simulink model "35 Bus Network Electricity Transmission Model"  (R2023b)
settings: Solver=VariableStepAuto  StartTime=0.0  StopTime=1  RelTol=1e-3
model workspace (MAT data in the model file):
  T_set = 0.0001
  Tp = 5e-05
undefined symbols (not defined in the file): D1, D11, Delta, DiscIntNeverNeededParam
libraries: spsSeriesRLCBranchLib x57, spsLoadFlowBusLib x35, spsThreePhaseSeriesRLCLoadLib x28, spsThreePhaseTransformerTwoWindingsLib x22, spsDistributedParametersLineLib x22, spsGenericPowerSystemStabilizerLib x20, spsThreePhaseVIMeasurementLib x14, spsSynchronousMachinepuStandardLib x10, spsExcitationSystemLib x10, spsHydraulicTurbineandGovernorLib x10, spsFourierLib x8, spsMeanLib x8
(part 7 of 8)

== system 35 Bus Network Electricity Transmission Model/400 kV Solar Farm/VSC Control/Current Regulator ==
  note: harmonic filter neglected
  note: Vd_mes + Id*R - Iq*L + deriv(Id)*L= Vd_conv
  note: Vq_mes + Id*L + Iq*R + deriv(Iq)*L= Vq_conv
  note: Current Regulator
      | (with feedforward)
  note: Sign Convention: Current going out of the converter = positive current
  note: Iq positive --> The converter absorbs reactive power ("Inductive mode") = Reactive Power Q negative
  note: Id positive --> The converter generates active power ("Inverter mode") = Active Power P positive
  note: Ltot = Lxfo + Lchoke
      | Rtot = Rxfo + Rchoke
  note: (Vd_prim - Vd_conv) ~= + Iq * Ltot
  note: (Vq_prim - Vq_conv) ~ = - Id * Ltot
  note: For Ltot >> Rtot :
  VdVq_mes : Inport  PortDimensions=2
  IdIq_mes : Inport  Port=2  PortDimensions=2
  IdIq_ref : Inport  Port=3  PortDimensions=2
  Add1 : Sum  Inputs=++-
  Add2 : Sum
  Add3 : Sum  Inputs=+++
  Demux : Demux  Outputs=2
  Demux1 : Demux  Outputs=2
  Ltot_pu1 : Gain  Gain=Ltot_pu  SaturateOnIntegerOverflow=on  OutDataTypeStr=Inherit: Same as input  ParamDataTypeStr=Inherit: Same as input
  Ltot_pu2 : Gain  Gain=Ltot_pu  SaturateOnIntegerOverflow=on  OutDataTypeStr=Inherit: Same as input  ParamDataTypeStr=Inherit: Same as input
  Mux : Mux  Inputs=2
  PI : slpidlib/PID Controller  Controller=PI  Form=Parallel  TimeDomain=Discrete-time  UseExternalTs=off  SampleTime=Ts  IntegratorMethod=Forward Euler  FilterMethod=Forward Euler  ControllerParametersSource=internal  P=Kp_Ireg  I=Ki_Ireg  UseKiTs=off  D=0  N=100  UseFilter=on  TunerSelectOption=Transfer Function Based (PID Tuner App)  InitialConditionSource=internal  InitialConditionForIntegrator=0  InitialConditionForFilter=0  DifferentiatorICPrevScaledInput=0  ExternalReset=none  TrackingMode=off  Kt=1  LimitOutput=on  SatLimitsSource=internal  UpperSaturationLimit=2  LowerSaturationLimit=-2  LinearizeAsGain=off  AntiWindupMode=none  Kb=1  LimitIntegrator=off  UpperIntegratorSaturationLimit=inf  LowerIntegratorSaturationLimit=-inf  POutMin=[]  POutMax=[]  IOutMin=[]  IOutMax=[]  DOutMin=[]  DOutMax=[]  NOutMin=[]  NOutMax=[]  SumOutMin=[]  SumOutMax=[]  SaturationOutMin=[]  SaturationOutMax=[]  PParamMin=[]  PParamMax=[]  IParamMin=[]  IParamMax=[]  DParamMin=[]  DParamMax=[]  NParamMin=[]  NParamMax=[]  KbParamMin=[]  KbParamMax=[]  KtParamMin=[]  KtParamMax=[]  KbOutMin=[]  KbOutMax=[]  KtOutMin=[]  KtOutMax=[]  IntegratorOutMin=[]  IntegratorOutMax=[]  FilterOutMin=[]  FilterOutMax=[]  SumI1OutMin=[]  SumI1OutMax=[]  SumI2OutMin=[]  SumI2OutMax=[]  SumI3OutMin=[]  SumI3OutMax=[]  SumI4OutMin=[]  SumI4OutMax=[]  SumDOutMin=[]  SumDOutMax=[]  DifferentiatorOutMin=[]  DifferentiatorOutMax=[]  FilterDiffOutCoefMin=[]  FilterDiffOutCoefMax=[]  ReciprocalOutMin=[]  ReciprocalOutMax=[]  SumDenOutMin=[]  SumDenOutMax=[]  SumNumOutMin=[]  SumNumOutMax=[]  DivideOutMin=[]  DivideOutMax=[]  UdiffTsProdOutMin=[]  UdiffTsProdOutMax=[]  NTsProdOutMin=[]  NTsProdOutMax=[]  UintegralTsProdOutMin=[]  UintegralTsProdOutMax=[]  UngainTsProdOutMin=[]  UngainTsProdOutMax=[]  ClampingZeroOutDataTypeStr=Inherit: Inherit via back propagation  ClampingZeroOutMin=[]  ClampingZeroOutMax=[]  FilterDenConstantOutDataTypeStr=Inherit: Inherit via back propagation  FilterDenConstantOutMin=[]  FilterDenConstantOutMax=[]  PCopyOutDataTypeStr=Inherit: Inherit via back propagation  PCopyOutMin=[]  PCopyOutMax=[]  NCopyOutDataTypeStr=Inherit: Inherit via back propagation  NCopyOutMin=[]  NCopyOutMax=[]  IntegratorContinuousStateAttributes=''  IntegratorStateMustResolveToSignalObject=off  IntegratorRTWStateStorageClass=Auto  FilterContinuousStateAttributes=''  FilterStateMustResolveToSignalObject=off  FilterRTWStateStorageClass=Auto  ParallelPVariant=InternalParameters  IdealPVariant=Disabled  IVariant=InternalParameters  DVariant=Disabled  IntegratorVariant=Discrete  SatVariant=Enabled  AWVariant=Passthrough  PCopyVariant=Disabled  TRVariant=Disabled  FdbkBlocksVariant=Forward  IdealPFdbkVariant=Disabled  SatFdbkVariant=Disabled  DerivativeFilterVariant=Disabled  NVariant=Disabled  NCopyVariant=Disabled_SignalSpec  FilterICVariant=Disabled  IntegratorICVariant=InternalICs  ExternalResetVariant=Disabled  TRSumVariant=Passthrough  SumFdbkVariant=Disabled  SumVariant=Sum_PI  TsampFilterVariant=InternalTs  TsampNgainVariant=Passthrough  TsampIntegralVariant=Disabled_SignalSpec  ExternalSaturationOutDataTypeStr=Inherit: Same as second input
  PI_Ireg1 : Scope
  Rtot_pu1 : Gain  Gain=Rtot_pu  SaturateOnIntegerOverflow=on  OutDataTypeStr=Inherit: Same as input  ParamDataTypeStr=Inherit: Same as input
  Rtot_pu5 : Gain  Gain=Rtot_pu  SaturateOnIntegerOverflow=on  OutDataTypeStr=Inherit: Same as input  ParamDataTypeStr=Inherit: Same as input
  Saturation : Saturate  UpperLimit=2  LowerLimit=-2
  Sum : Sum  Inputs=|-+
  VdVq_conv : Outport  VectorParamsAs1DForOutWhenUnconnected=off
  wires:
  Mux/1 -> PI_Ireg1/1, Add2/2
  PI/1 -> Add2/1  "PI"
  Sum/1 -> PI/1
  IdIq_ref/1 -> Sum/2, Demux1/1
  IdIq_mes/1 -> Sum/1
  Add2/1 -> Saturation/1
  Saturation/1 -> VdVq_conv/1
  VdVq_mes/1 -> Demux/1
  Demux/1 -> Add1/1
  Rtot_pu1/1 -> Add1/2
  Demux1/1 -> Rtot_pu1/1, Ltot_pu2/1
  Ltot_pu1/1 -> Add1/3
  Demux1/2 -> Ltot_pu1/1, Rtot_pu5/1
  Rtot_pu5/1 -> Add3/2
  Ltot_pu2/1 -> Add3/3
  Add1/1 -> Mux/1  "Feedforward"
  Demux/2 -> Add3/1
  Add3/1 -> Mux/2

== system 35 Bus Network Electricity Transmission Model/400 kV Solar Farm/VSC Control/PLL & Measurements ==
  Vabc_prim : Inport
  Iabc_prim : Inport  Port=2
  PLL (3ph) : spsPLL3phLib/PLL (3ph)  Fmin=45  Par_Init="[-0.57  Fnom]"  ParK=[180, 3200, 1]  TcD=Ts  MaxRateChangeFreq=12  FilterCutOffFreq=25  Ts=Ts  AGC=on
  Selector1 : Selector  InputPortWidth=3  IndexOptions=Index vector (dialog)  Indices=[1 2]  OutputSizes=1
  Selector2 : Selector  InputPortWidth=3  IndexOptions=Index vector (dialog)  Indices=[1 2]  OutputSizes=1
  Terminator : Terminator
  V->pu : Gain  Gain=1/(Vnom_prim*sqrt(2)/sqrt(3))  SaturateOnIntegerOverflow=on  OutDataTypeStr=Inherit: Same as input  ParamDataTypeStr=Inherit: Same as input
  V->pu1 : Gain  Gain=Vnom_prim*sqrt(3)/Pnom/sqrt(2)  SaturateOnIntegerOverflow=on  OutDataTypeStr=Inherit: Same as input  ParamDataTypeStr=Inherit: Same as input
  abc to dq0 : spsabctodq0Lib/abc to dq0  Alignment=90 degrees behind phase A axis
  abc to dq1 : spsabctodq0Lib/abc to dq0  Alignment=90 degrees behind phase A axis
  wt : Outport  VectorParamsAs1DForOutWhenUnconnected=off
  VdVq_prim : Outport  Port=2  VectorParamsAs1DForOutWhenUnconnected=off
  IdIq_prim : Outport  Port=3  VectorParamsAs1DForOutWhenUnconnected=off
  wires:
  V->pu1/1 -> abc to dq1/1
  V->pu/1 -> PLL (3ph)/1, abc to dq0/1
  abc to dq1/1 -> Selector1/1
  Vabc_prim/1 -> V->pu/1
  Iabc_prim/1 -> V->pu1/1
  abc to dq0/1 -> Selector2/1
  Selector2/1 -> VdVq_prim/1
  Selector1/1 -> IdIq_prim/1
  PLL (3ph)/2 -> wt/1, abc to dq1/2, abc to dq0/2
  PLL (3ph)/1 -> Terminator/1

== system 35 Bus Network Electricity Transmission Model/400 kV Solar Farm/VSC Control/Uabc_ref Generation max (m) = 1 ==
  note: (Correction for transformer
      |  D1 connection)
  note: (Correction for delai of Ts_Control)
  wt : Inport
  VdVq_conv : Inport  Port=2
  Add1 : Sum  Inputs=++++
  Add2 : Sum
  Complex to Magnitude-Angle : ComplexToMagnitudeAngle
  Constant : Constant  Value=-pi/6
  Constant1 : Constant  Value=Vnom_dc
  Constant2 : Constant  Value="[ 0  -2*pi/3  2*pi/3  ]"
  Constant3 : Constant  Value=Vnom_sec*sqrt(2)/sqrt(3)
  Constant4 : Constant  Value=Ts*Fnom*(2*pi)
  Demux1 : Demux  Outputs=2
  Gain1 : Gain  Gain=1/2
  Product : Product  Inputs=*/  RndMeth=Zero
  Product1 : Product  Inputs=*/  RndMeth=Zero
  Product2 : Product  Inputs=**  RndMeth=Zero
  Real-Imag to Complex : RealImagToComplex
  Saturation : Saturate  UpperLimit=1  LowerLimit=0
  Trigonometric Function : Trigonometry
  Uabc_ref : Outport  VectorParamsAs1DForOutWhenUnconnected=off
  wires:
  Complex to Magnitude-Angle/1 -> Saturation/1
  Constant1/1 -> Gain1/1
  VdVq_conv/1 -> Product1/1
  Product1/1 -> Demux1/1
  Gain1/1 -> Product/1
  Real-Imag to Complex/1 -> Complex to Magnitude-Angle/1
  Demux1/1 -> Real-Imag to Complex/1
  Demux1/2 -> Real-Imag to Complex/2
  Constant2/1 -> Add1/2
  Constant/1 -> Add1/3
  Constant3/1 -> Product/2
  Product/1 -> Product1/2
  Complex to Magnitude-Angle/2 -> Add2/1
  Add1/1 -> Add2/2
  Add2/1 -> Trigonometric Function/1
  Saturation/1 -> Product2/1
  Trigonometric Function/1 -> Product2/2
  Product2/1 -> Uabc_ref/1
  wt/1 -> Add1/1
  Constant4/1 -> Add1/4

== system 35 Bus Network Electricity Transmission Model/400 kV Solar Farm/VSC Control/VDC Regulator ==
  Vdc_mes : Inport  PortDimensions=1
  Vdc_ref : Inport  Port=2  PortDimensions=1
  PI : slpidlib/PID Controller  Controller=PI  Form=Parallel  TimeDomain=Discrete-time  UseExternalTs=off  SampleTime=Ts  IntegratorMethod=Trapezoidal  FilterMethod=Forward Euler  ControllerParametersSource=internal  P=Kp_VDCreg  I=Ki_VDCreg  UseKiTs=off  D=0  N=100  UseFilter=on  TunerSelectOption=Transfer Function Based (PID Tuner App)  InitialConditionSource=internal  InitialConditionForIntegrator=0  InitialConditionForFilter=0  DifferentiatorICPrevScaledInput=0  ExternalReset=none  TrackingMode=off  Kt=1  LimitOutput=on  SatLimitsSource=internal  UpperSaturationLimit=1.5  LowerSaturationLimit=-1.5  LinearizeAsGain=off  AntiWindupMode=none  Kb=1  LimitIntegrator=off  UpperIntegratorSaturationLimit=inf  LowerIntegratorSaturationLimit=-inf  POutMin=[]  POutMax=[]  IOutMin=[]  IOutMax=[]  DOutMin=[]  DOutMax=[]  NOutMin=[]  NOutMax=[]  SumOutMin=[]  SumOutMax=[]  SaturationOutMin=[]  SaturationOutMax=[]  PParamMin=[]  PParamMax=[]  IParamMin=[]  IParamMax=[]  DParamMin=[]  DParamMax=[]  NParamMin=[]  NParamMax=[]  KbParamMin=[]  KbParamMax=[]  KtParamMin=[]  KtParamMax=[]  KbOutMin=[]  KbOutMax=[]  KtOutMin=[]  KtOutMax=[]  IntegratorOutMin=[]  IntegratorOutMax=[]  FilterOutMin=[]  FilterOutMax=[]  SumI1OutMin=[]  SumI1OutMax=[]  SumI2OutMin=[]  SumI2OutMax=[]  SumI3OutMin=[]  SumI3OutMax=[]  SumI4OutMin=[]  SumI4OutMax=[]  SumDOutMin=[]  SumDOutMax=[]  DifferentiatorOutMin=[]  DifferentiatorOutMax=[]  FilterDiffOutCoefMin=[]  FilterDiffOutCoefMax=[]  ReciprocalOutMin=[]  ReciprocalOutMax=[]  SumDenOutMin=[]  SumDenOutMax=[]  SumNumOutMin=[]  SumNumOutMax=[]  DivideOutMin=[]  DivideOutMax=[]  UdiffTsProdOutMin=[]  UdiffTsProdOutMax=[]  NTsProdOutMin=[]  NTsProdOutMax=[]  UintegralTsProdOutMin=[]  UintegralTsProdOutMax=[]  UngainTsProdOutMin=[]  UngainTsProdOutMax=[]  ClampingZeroOutDataTypeStr=Inherit: Inherit via back propagation  ClampingZeroOutMin=[]  ClampingZeroOutMax=[]  FilterDenConstantOutDataTypeStr=Inherit: Inherit via back propagation  FilterDenConstantOutMin=[]  FilterDenConstantOutMax=[]  PCopyOutDataTypeStr=Inherit: Inherit via back propagation  PCopyOutMin=[]  PCopyOutMax=[]  NCopyOutDataTypeStr=Inherit: Inherit via back propagation  NCopyOutMin=[]  NCopyOutMax=[]  IntegratorContinuousStateAttributes=''  IntegratorStateMustResolveToSignalObject=off  IntegratorRTWStateStorageClass=Auto  FilterContinuousStateAttributes=''  FilterStateMustResolveToSignalObject=off  FilterRTWStateStorageClass=Auto  ParallelPVariant=InternalParameters  IdealPVariant=Disabled  IVariant=InternalParameters  DVariant=Disabled  IntegratorVariant=Discrete  SatVariant=Enabled  AWVariant=Passthrough  PCopyVariant=Disabled  TRVariant=Disabled  FdbkBlocksVariant=Forward  IdealPFdbkVariant=Disabled  SatFdbkVariant=Disabled  DerivativeFilterVariant=Disabled  NVariant=Disabled  NCopyVariant=Disabled_SignalSpec  FilterICVariant=Disabled  IntegratorICVariant=InternalICs  ExternalResetVariant=Disabled  TRSumVariant=Passthrough  SumFdbkVariant=Disabled  SumVariant=Sum_PI  TsampFilterVariant=InternalTs  TsampNgainVariant=Passthrough  TsampIntegralVariant=Disabled_SignalSpec  ExternalSaturationOutDataTypeStr=Inherit: Same as second input
  Rtot_pu3 : Gain  Gain=1/Vnom_dc  SaturateOnIntegerOverflow=on  OutDataTypeStr=Inherit: Same as input  ParamDataTypeStr=Inherit: Same as input
  Sum : Sum  Inputs=|+-
  Id_ref : Outport  SampleTime=Ts  InitialOutput=0  VectorParamsAs1DForOutWhenUnconnected=off
  wires:
  Sum/1 -> Rtot_pu3/1
  Vdc_mes/1 -> Sum/1
  Vdc_ref/1 -> Sum/2
  Rtot_pu3/1 -> PI/1
  PI/1 -> Id_ref/1

== system 35 Bus Network Electricity Transmission Model/North Network/Regulators 7/Turbine and Excitation Regulators ==
  pref : Inport
  w : Inport  Port=2
  Pe 0 : Inport  Port=3
  Vref : Inport  Port=4
  Vm : Inport  Port=5
  Add : Sum  Inputs=+-
  Complex to Real-Imag : ComplexToRealImag
  Excitation System : spsExcitationSystemLib/Excitation System  tr=20e-3  reg=[ 300, 0.001 ]  exc=[ 1, 0 ]  tgr=[ 0, 0 ]  damp=[ 0.001, 0.1 ]  sat=[ 0, 0 ]  lim=[ -11.5, 11.5, 0 ]  v0="[1.0  1.28]"
      settings: LibrarySourceBlock=sps_lib/Electrical Machines/Synchronous Machine Control/Excitation System
  Hydraulic Turbine and Governor : spsHydraulicTurbineandGovernorLib/Hydraulic Turbine and Governor  sm="[ 10/3  0.07 ]"  gate="[  0.01  0.97518  -0.1  0.1 ]"  reg="[  0.05  1.163  0.105  0  0.01  ]"  hyd="[  0  2.67  ]"  dref=0  po=0.7516
      settings: LibrarySourceBlock=|
      | sps_lib/Electrical Machines/Synchronous Machine Control/Hydraulic Turbine
      | and Governor
  Stabilitator : Subsystem
  Terminator : Terminator
  wref : Constant
  wref1 : Constant
  Pm : Outport
  Vf : Outport  Port=2
  wires:
  pref/1 -> Hydraulic Turbine and Governor/2
  Complex to Real-Imag/2 -> Excitation System/3
  wref/1 -> Hydraulic Turbine and Governor/1
  Add/1 -> Stabilitator/3(dw), Hydraulic Turbine and Governor/5
  Vm/1 -> Complex to Real-Imag/1
  Pe 0/1 -> Stabilitator/2(Pe), Hydraulic Turbine and Governor/4
  Hydraulic Turbine and Governor/2 -> Terminator/1
  Stabilitator/1(Out1) -> Excitation System/4
  w/1 -> Add/1, Hydraulic Turbine and Governor/3
  Excitation System/1 -> Vf/1
  Hydraulic Turbine and Governor/1 -> Pm/1, Stabilitator/1(Pm)
  Vref/1 -> Excitation System/1
  wref1/1 -> Add/2
  Complex to Real-Imag/1 -> Excitation System/2

== system 35 Bus Network Electricity Transmission Model/North Network/Regulators 8/Turbine and Excitation Regulators ==
  pref : Inport
  w : Inport  Port=2
  Pe 0 : Inport  Port=3
  Vref : Inport  Port=4
  Vm : Inport  Port=5
  Add : Sum  Inputs=+-
  Complex to Real-Imag : ComplexToRealImag
  Excitation System : spsExcitationSystemLib/Excitation System  tr=20e-3  reg=[ 300, 0.001 ]  exc=[ 1, 0 ]  tgr=[ 0, 0 ]  damp=[ 0.001, 0.1 ]  sat=[ 0, 0 ]  lim=[ -11.5, 11.5, 0 ]  v0="[1.0  1.28]"
      settings: LibrarySourceBlock=sps_lib/Electrical Machines/Synchronous Machine Control/Excitation System
  Hydraulic Turbine and Governor : spsHydraulicTurbineandGovernorLib/Hydraulic Turbine and Governor  sm="[ 10/3  0.07 ]"  gate="[  0.01  0.97518  -0.1  0.1 ]"  reg="[  0.05  1.163  0.105  0  0.01  ]"  hyd="[  0  2.67  ]"  dref=0  po=0.7516
      settings: LibrarySourceBlock=|
      | sps_lib/Electrical Machines/Synchronous Machine Control/Hydraulic Turbine
      | and Governor
  Stabilitator : Subsystem
  Terminator : Terminator
  wref : Constant
  wref1 : Constant
  Pm : Outport
  Vf : Outport  Port=2
  wires:
  pref/1 -> Hydraulic Turbine and Governor/2
  Complex to Real-Imag/2 -> Excitation System/3
  wref/1 -> Hydraulic Turbine and Governor/1
  Add/1 -> Stabilitator/3(dw), Hydraulic Turbine and Governor/5
  Vm/1 -> Complex to Real-Imag/1
  Pe 0/1 -> Stabilitator/2(Pe), Hydraulic Turbine and Governor/4
  Hydraulic Turbine and Governor/2 -> Terminator/1
  Stabilitator/1(Out1) -> Excitation System/4
  w/1 -> Add/1, Hydraulic Turbine and Governor/3
  Excitation System/1 -> Vf/1
  Hydraulic Turbine and Governor/1 -> Pm/1, Stabilitator/1(Pm)
  Vref/1 -> Excitation System/1
  wref1/1 -> Add/2
  Complex to Real-Imag/1 -> Excitation System/2

== system 35 Bus Network Electricity Transmission Model/North Network/Regulators 9/Turbine and Excitation Regulators ==
  pref : Inport
  w : Inport  Port=2
  Pe 0 : Inport  Port=3
  Vref : Inport  Port=4
  Vm : Inport  Port=5
  Add : Sum  Inputs=+-
  Complex to Real-Imag : ComplexToRealImag
  Excitation System : spsExcitationSystemLib/Excitation System  tr=20e-3  reg=[ 300, 0.001 ]  exc=[ 1, 0 ]  tgr=[ 0, 0 ]  damp=[ 0.001, 0.1 ]  sat=[ 0, 0 ]  lim=[ -11.5, 11.5, 0 ]  v0="[1.0  1.28]"
      settings: LibrarySourceBlock=sps_lib/Electrical Machines/Synchronous Machine Control/Excitation System
  Hydraulic Turbine and Governor : spsHydraulicTurbineandGovernorLib/Hydraulic Turbine and Governor  sm="[ 10/3  0.07 ]"  gate="[  0.01  0.97518  -0.1  0.1 ]"  reg="[  0.05  1.163  0.105  0  0.01  ]"  hyd="[  0  2.67  ]"  dref=0  po=0.7516
      settings: LibrarySourceBlock=|
      | sps_lib/Electrical Machines/Synchronous Machine Control/Hydraulic Turbine
      | and Governor
  Stabilitator : Subsystem
  Terminator : Terminator
  wref : Constant
  wref1 : Constant
  Pm : Outport
  Vf : Outport  Port=2
  wires:
  pref/1 -> Hydraulic Turbine and Governor/2
  Complex to Real-Imag/2 -> Excitation System/3
  wref/1 -> Hydraulic Turbine and Governor/1
  Add/1 -> Stabilitator/3(dw), Hydraulic Turbine and Governor/5
  Vm/1 -> Complex to Real-Imag/1
  Pe 0/1 -> Stabilitator/2(Pe), Hydraulic Turbine and Governor/4
  Hydraulic Turbine and Governor/2 -> Terminator/1
  Stabilitator/1(Stab) -> Excitation System/4
  w/1 -> Add/1, Hydraulic Turbine and Governor/3
  Excitation System/1 -> Vf/1
  Hydraulic Turbine and Governor/1 -> Pm/1, Stabilitator/1(Pm)
  Vref/1 -> Excitation System/1
  wref1/1 -> Add/2
  Complex to Real-Imag/1 -> Excitation System/2

== system 35 Bus Network Electricity Transmission Model/Regulators 10/Turbine and Excitation Regulators/Stabilitator ==
  Pm : Inport
  Pe : Inport  Port=2
  dw : Inport  Port=3
  Add1 : Sum  Inputs=+-
  Generic Power System Stabilizer : spsGenericPowerSystemStabilizerLib/Generic Power System Stabilizer  Tsensor=30e-3  K=20  Twashout=2  Tleadlag1=[50e-3 20e-3]  Tleadlag2=[3 5.4]  VSlimits=[-0.15 0.15]  Vinit=0  Plot_On=off  MagdB_On=on  FreqRange=logspace(-2,2,500)
      settings: LibrarySourceBlock=|
      | sps_lib/Electrical Machines/Synchronous Machine Control/Generic
      | Power System Stabilizer
  Generic Power System Stabilizer1 : spsGenericPowerSystemStabilizerLib/Generic Power System Stabilizer  Tsensor=30e-3  K=20  Twashout=2  Tleadlag1=[50e-3 20e-3]  Tleadlag2=[3 5.4]  VSlimits=[-0.15 0.15]  Vinit=0  Plot_On=off  MagdB_On=on  FreqRange=logspace(-2,2,500)
      settings: LibrarySourceBlock=|
      | sps_lib/Electrical Machines/Synchronous Machine Control/Generic
      | Power System Stabilizer
  Ground : Ground
  Multiport Switch : MultiPortSwitch  DiagnosticForDefault=None  SaturateOnIntegerOverflow=off  InputSameDT=off
  Out1 : Outport
  wires:
  Pm/1 -> Add1/1
  Generic Power System Stabilizer1/1 -> Multiport Switch/4
  Pe/1 -> Add1/2
  Add1/1 -> Generic Power System Stabilizer/1
  Generic Power System Stabilizer/1 -> Multiport Switch/3
  dw/1 -> Generic Power System Stabilizer1/1
  Ground/1 -> Multiport Switch/2
  [PSS_modes] -> Multiport Switch/1
  Multiport Switch/1 -> Out1/1

== system 35 Bus Network Electricity Transmission Model/South Network/Regulators 1/Turbine and Excitation Regulators ==
  pref : Inport
  w : Inport  Port=2
  Pe 0 : Inport  Port=3
  Vref : Inport  Port=4
  Vm : Inport  Port=5
  Add : Sum  Inputs=+-
  Complex to Real-Imag : ComplexToRealImag
  Excitation System : spsExcitationSystemLib/Excitation System  tr=20e-3  reg=[ 300, 0.001 ]  exc=[ 1, 0 ]  tgr=[ 0, 0 ]  damp=[ 0.001, 0.1 ]  sat=[ 0, 0 ]  lim=[ -11.5, 11.5, 0 ]  v0="[1.0  1.28]"
      settings: LibrarySourceBlock=sps_lib/Electrical Machines/Synchronous Machine Control/Excitation System
  Hydraulic Turbine and Governor : spsHydraulicTurbineandGovernorLib/Hydraulic Turbine and Governor  sm="[ 10/3  0.07 ]"  gate="[  0.01  0.97518  -0.1  0.1 ]"  reg="[  0.05  1.163  0.105  0  0.01  ]"  hyd="[  0  2.67  ]"  dref=0  po=0.7516
      settings: LibrarySourceBlock=|
      | sps_lib/Electrical Machines/Synchronous Machine Control/Hydraulic Turbine
      | and Governor
  Stabilitator : Subsystem
  Terminator : Terminator
  wref : Constant
  wref1 : Constant
  Pm : Outport
  Vf : Outport  Port=2
  wires:
  pref/1 -> Hydraulic Turbine and Governor/2
  Complex to Real-Imag/2 -> Excitation System/3
  wref/1 -> Hydraulic Turbine and Governor/1
  Add/1 -> Stabilitator/3(dw), Hydraulic Turbine and Governor/5
  Vm/1 -> Complex to Real-Imag/1
  Pe 0/1 -> Stabilitator/2(Pe), Hydraulic Turbine and Governor/4
  Hydraulic Turbine and Governor/2 -> Terminator/1
  Stabilitator/1(Out1) -> Excitation System/4
  w/1 -> Add/1, Hydraulic Turbine and Governor/3
  Excitation System/1 -> Vf/1
  Hydraulic Turbine and Governor/1 -> Pm/1, Stabilitator/1(Pm)
  Vref/1 -> Excitation System/1
  wref1/1 -> Add/2
  Complex to Real-Imag/1 -> Excitation System/2

== system 35 Bus Network Electricity Transmission Model/South Network/Regulators 2/Turbine and Excitation Regulators ==
  pref : Inport
  w : Inport  Port=2
  Pe 0 : Inport  Port=3
  Vref : Inport  Port=4
  Vm : Inport  Port=5
  Add : Sum  Inputs=+-
  Complex to Real-Imag : ComplexToRealImag
  Excitation System : spsExcitationSystemLib/Excitation System  tr=20e-3  reg=[ 300, 0.001 ]  exc=[ 1, 0 ]  tgr=[ 0, 0 ]  damp=[ 0.001, 0.1 ]  sat=[ 0, 0 ]  lim=[ -11.5, 11.5, 0 ]  v0="[1.0  1.28]"
      settings: LibrarySourceBlock=sps_lib/Electrical Machines/Synchronous Machine Control/Excitation System
  Hydraulic Turbine and Governor : spsHydraulicTurbineandGovernorLib/Hydraulic Turbine and Governor  sm="[ 10/3  0.07 ]"  gate="[  0.01  0.97518  -0.1  0.1 ]"  reg="[  0.05  1.163  0.105  0  0.01  ]"  hyd="[  0  2.67  ]"  dref=0  po=0.7516
      settings: LibrarySourceBlock=|
      | sps_lib/Electrical Machines/Synchronous Machine Control/Hydraulic Turbine
      | and Governor
  Stabilitator : Subsystem
  Terminator : Terminator
  wref : Constant
  wref1 : Constant
  Pm : Outport
  Vf : Outport  Port=2
  wires:
  pref/1 -> Hydraulic Turbine and Governor/2
  Complex to Real-Imag/2 -> Excitation System/3
  wref/1 -> Hydraulic Turbine and Governor/1
  Add/1 -> Stabilitator/3(dw), Hydraulic Turbine and Governor/5
  Vm/1 -> Complex to Real-Imag/1
  Pe 0/1 -> Stabilitator/2(Pe), Hydraulic Turbine and Governor/4
  Hydraulic Turbine and Governor/2 -> Terminator/1
  Stabilitator/1(Out1) -> Excitation System/4
  w/1 -> Add/1, Hydraulic Turbine and Governor/3
  Excitation System/1 -> Vf/1
  Hydraulic Turbine and Governor/1 -> Pm/1, Stabilitator/1(Pm)
  Vref/1 -> Excitation System/1
  wref1/1 -> Add/2
  Complex to Real-Imag/1 -> Excitation System/2

== system 35 Bus Network Electricity Transmission Model/South Network/Regulators 3/Turbine and Excitation Regulators ==
  pref : Inport
  w : Inport  Port=2
  Pe 0 : Inport  Port=3
  Vref : Inport  Port=4
  Vm : Inport  Port=5
  Add : Sum  Inputs=+-
  Complex to Real-Imag : ComplexToRealImag
  Excitation System : spsExcitationSystemLib/Excitation System  tr=20e-3  reg=[ 300, 0.001 ]  exc=[ 1, 0 ]  tgr=[ 0, 0 ]  damp=[ 0.001, 0.1 ]  sat=[ 0, 0 ]  lim=[ -11.5, 11.5, 0 ]  v0="[1.0  1.28]"
      settings: LibrarySourceBlock=sps_lib/Electrical Machines/Synchronous Machine Control/Excitation System
  Hydraulic Turbine and Governor : spsHydraulicTurbineandGovernorLib/Hydraulic Turbine and Governor  sm="[ 10/3  0.07 ]"  gate="[  0.01  0.97518  -0.1  0.1 ]"  reg="[  0.05  1.163  0.105  0  0.01  ]"  hyd="[  0  2.67  ]"  dref=0  po=0.7516
      settings: LibrarySourceBlock=|
      | sps_lib/Electrical Machines/Synchronous Machine Control/Hydraulic Turbine
      | and Governor
  Stabilitator : Subsystem
  Terminator : Terminator
  wref : Constant
  wref1 : Constant
  Pm : Outport
  Vf : Outport  Port=2
  wires:
  pref/1 -> Hydraulic Turbine and Governor/2
  Complex to Real-Imag/2 -> Excitation System/3
  wref/1 -> Hydraulic Turbine and Governor/1
  Add/1 -> Stabilitator/3(dw), Hydraulic Turbine and Governor/5
  Vm/1 -> Complex to Real-Imag/1
  Pe 0/1 -> Stabilitator/2(Pe), Hydraulic Turbine and Governor/4
  Hydraulic Turbine and Governor/2 -> Terminator/1
  Stabilitator/1(Out1) -> Excitation System/4
  w/1 -> Add/1, Hydraulic Turbine and Governor/3
  Excitation System/1 -> Vf/1
  Hydraulic Turbine and Governor/1 -> Pm/1, Stabilitator/1(Pm)
  Vref/1 -> Excitation System/1
  wref1/1 -> Add/2
  Complex to Real-Imag/1 -> Excitation System/2

== system 35 Bus Network Electricity Transmission Model/South Network/Regulators 4/Turbine and Excitation Regulators ==
  pref : Inport
  w : Inport  Port=2
  Pe 0 : Inport  Port=3
  Vref : Inport  Port=4
  Vm : Inport  Port=5
  Add : Sum  Inputs=+-
  Complex to Real-Imag : ComplexToRealImag
  Excitation System : spsExcitationSystemLib/Excitation System  tr=20e-3  reg=[ 300, 0.001 ]  exc=[ 1, 0 ]  tgr=[ 0, 0 ]  damp=[ 0.001, 0.1 ]  sat=[ 0, 0 ]  lim=[ -11.5, 11.5, 0 ]  v0="[1.0  1.28]"
      settings: LibrarySourceBlock=sps_lib/Electrical Machines/Synchronous Machine Control/Excitation System
  Hydraulic Turbine and Governor : spsHydraulicTurbineandGovernorLib/Hydraulic Turbine and Governor  sm="[ 10/3  0.07 ]"  gate="[  0.01  0.97518  -0.1  0.1 ]"  reg="[  0.05  1.163  0.105  0  0.01  ]"  hyd="[  0  2.67  ]"  dref=0  po=0.7516
      settings: LibrarySourceBlock=|
      | sps_lib/Electrical Machines/Synchronous Machine Control/Hydraulic Turbine
      | and Governor
  Stabilitator : Subsystem
  Terminator : Terminator
  wref : Constant
  wref1 : Constant
  Pm : Outport
  Vf : Outport  Port=2
  wires:
  pref/1 -> Hydraulic Turbine and Governor/2
  Complex to Real-Imag/2 -> Excitation System/3
  wref/1 -> Hydraulic Turbine and Governor/1
  Add/1 -> Hydraulic Turbine and Governor/5, Stabilitator/3(dw)
  Vm/1 -> Complex to Real-Imag/1
  Pe 0/1 -> Stabilitator/2(Pe), Hydraulic Turbine and Governor/4
  Hydraulic Turbine and Governor/2 -> Terminator/1
  Stabilitator/1(Out1) -> Excitation System/4
  w/1 -> Add/1, Hydraulic Turbine and Governor/3
  Excitation System/1 -> Vf/1
  Hydraulic Turbine and Governor/1 -> Pm/1, Stabilitator/1(Pm)
  Vref/1 -> Excitation System/1
  wref1/1 -> Add/2
  Complex to Real-Imag/1 -> Excitation System/2

== system 35 Bus Network Electricity Transmission Model/South Network/Regulators 5/Turbine and Excitation Regulators ==
  pref : Inport
  w : Inport  Port=2
  Pe 0 : Inport  Port=3
  Vref : Inport  Port=4
  Vm : Inport  Port=5
  Add : Sum  Inputs=+-
  Complex to Real-Imag : ComplexToRealImag
  Excitation System : spsExcitationSystemLib/Excitation System  tr=20e-3  reg=[ 300, 0.001 ]  exc=[ 1, 0 ]  tgr=[ 0, 0 ]  damp=[ 0.001, 0.1 ]  sat=[ 0, 0 ]  lim=[ -11.5, 11.5, 0 ]  v0="[1.0  1.28]"
      settings: LibrarySourceBlock=sps_lib/Electrical Machines/Synchronous Machine Control/Excitation System
  Hydraulic Turbine and Governor : spsHydraulicTurbineandGovernorLib/Hydraulic Turbine and Governor  sm="[ 10/3  0.07 ]"  gate="[  0.01  0.97518  -0.1  0.1 ]"  reg="[  0.05  1.163  0.105  0  0.01  ]"  hyd="[  0  2.67  ]"  dref=0  po=0.7516
      settings: LibrarySourceBlock=|
      | sps_lib/Electrical Machines/Synchronous Machine Control/Hydraulic Turbine
      | and Governor
  Stabilitator : Subsystem
  Terminator : Terminator
  wref : Constant
  wref1 : Constant
  Pm : Outport
  Vf : Outport  Port=2
  wires:
  pref/1 -> Hydraulic Turbine and Governor/2
  Complex to Real-Imag/2 -> Excitation System/3
  wref/1 -> Hydraulic Turbine and Governor/1
  Add/1 -> Stabilitator/3(dw), Hydraulic Turbine and Governor/5
  Vm/1 -> Complex to Real-Imag/1
  Pe 0/1 -> Stabilitator/2(Pe), Hydraulic Turbine and Governor/4
  Hydraulic Turbine and Governor/2 -> Terminator/1
  Stabilitator/1(Out1) -> Excitation System/4
  w/1 -> Add/1, Hydraulic Turbine and Governor/3
  Excitation System/1 -> Vf/1
  Hydraulic Turbine and Governor/1 -> Pm/1, Stabilitator/1(Pm)
  Vref/1 -> Excitation System/1
  wref1/1 -> Add/2
  Complex to Real-Imag/1 -> Excitation System/2

== system 35 Bus Network Electricity Transmission Model/South Network/Regulators 6/Turbine and Excitation Regulators ==
  pref : Inport
  w : Inport  Port=2
  Pe 0 : Inport  Port=3
  Vref : Inport  Port=4
  Vm : Inport  Port=5
  Add : Sum  Inputs=+-
  Complex to Real-Imag : ComplexToRealImag
  Excitation System : spsExcitationSystemLib/Excitation System  tr=20e-3  reg=[ 300, 0.001 ]  exc=[ 1, 0 ]  tgr=[ 0, 0 ]  damp=[ 0.001, 0.1 ]  sat=[ 0, 0 ]  lim=[ -11.5, 11.5, 0 ]  v0="[1.0  1.28]"
      settings: LibrarySourceBlock=sps_lib/Electrical Machines/Synchronous Machine Control/Excitation System
  Hydraulic Turbine and Governor : spsHydraulicTurbineandGovernorLib/Hydraulic Turbine and Governor  sm="[ 10/3  0.07 ]"  gate="[  0.01  0.97518  -0.1  0.1 ]"  reg="[  0.05  1.163  0.105  0  0.01  ]"  hyd="[  0  2.67  ]"  dref=0  po=0.7516
      settings: LibrarySourceBlock=|
      | sps_lib/Electrical Machines/Synchronous Machine Control/Hydraulic Turbine
      | and Governor
  Stabilitator : Subsystem
  Terminator : Terminator
  wref : Constant
  wref1 : Constant
  Pm : Outport
  Vf : Outport  Port=2
  wires:
  pref/1 -> Hydraulic Turbine and Governor/2
  Complex to Real-Imag/2 -> Excitation System/3
  wref/1 -> Hydraulic Turbine and Governor/1
  Add/1 -> Stabilitator/3(dw), Hydraulic Turbine and Governor/5
  Vm/1 -> Complex to Real-Imag/1
  Pe 0/1 -> Stabilitator/2(Pe), Hydraulic Turbine and Governor/4
  Hydraulic Turbine and Governor/2 -> Terminator/1
  Stabilitator/1(Out1) -> Excitation System/4
  w/1 -> Add/1, Hydraulic Turbine and Governor/3
  Excitation System/1 -> Vf/1
  Hydraulic Turbine and Governor/1 -> Pm/1, Stabilitator/1(Pm)
  Vref/1 -> Excitation System/1
  wref1/1 -> Add/2
  Complex to Real-Imag/1 -> Excitation System/2

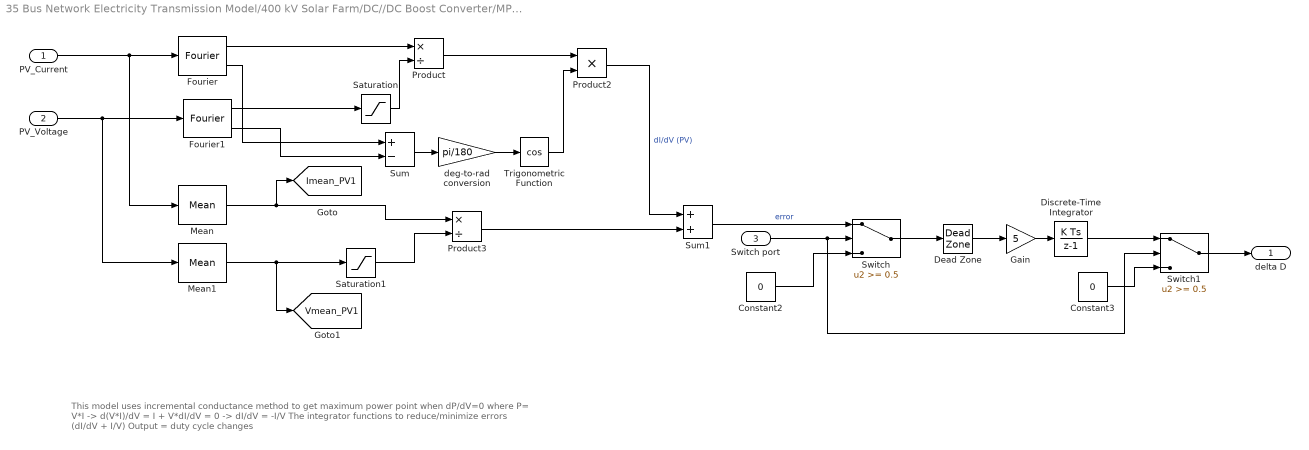
== system 35 Bus Network Electricity Transmission Model/400 kV Solar Farm/DC//DC Boost Converter/MPPT/MPPT  ==
  note: This model uses incremental conductance method to get maximum power point
      |
      | when dP/dV=0  where P= V*I
      | -> d(V*I)/dV = I + V*dI/dV = 0
      | -> dI/dV = -I/V
      |
      | The integrator functions to reduce/minimize errors (dI/dV + I/V)
      | Output = duty cycle changes
  PV_Current : Inport
  PV_Voltage : Inport  Port=2
  Switch port : Inport  Port=3
  Constant2 : Constant  Value=0
  Constant3 : Constant  Value=0
  Dead Zone : DeadZone  LowerValue=-0.05  UpperValue=0.05
  Discrete-Time Integrator : DiscreteIntegrator  SampleTime=T_set  LimitOutput=on  UpperSaturationLimit=1  LowerSaturationLimit=-1  ICPrevOutput=DiscIntNeverNeededParam  ICPrevScaledInput=DiscIntNeverNeededParam
  Fourier : spsFourierLib/Fourier  Freq=1/(MPPT_time)  n=1  InInit=[0, 0]  Ts=T_set
  Fourier1 : spsFourierLib/Fourier  Freq=1/(MPPT_time)  n=1  InInit=[0, 0]  Ts=T_set
  Gain : Gain  Gain=5
  Mean : spsMeanLib/Mean  Freq=1/(MPPT_time)  Vinit=0  Ts=T_set
  Mean1 : spsMeanLib/Mean  Freq=1/(MPPT_time)  Vinit=0  Ts=T_set
  Product : Product  Inputs=*/
  Product2 : Product
  Product3 : Product  Inputs=*/
  Saturation : Saturate  UpperLimit=inf  LowerLimit=eps  ZeroCross=off
  Saturation1 : Saturate  UpperLimit=inf  LowerLimit=eps  ZeroCross=off
  Sum : Sum  Inputs=+-
  Sum1 : Sum
  Switch : Switch  Threshold=0.5  SaturateOnIntegerOverflow=off  InputSameDT=off
  Switch1 : Switch  Threshold=0.5  SaturateOnIntegerOverflow=off  InputSameDT=off
  Trigonometric Function : Trigonometry  Operator=cos
  deg-to-rad conversion : Gain  Gain=pi/180
  delta D : Outport
  tag scope: Imean_PV1=global, Vmean_PV1=global
  wires:
  Mean1/1 -> [Vmean_PV1], Saturation1/1
  PV_Voltage/1 -> Mean1/1, Fourier1/1
  Sum/1 -> deg-to-rad conversion/1
  Product/1 -> Product2/1
  Product3/1 -> Sum1/2
  Saturation1/1 -> Product3/2
  Switch port/1 -> Switch/2, Switch1/2
  Mean/1 -> [Imean_PV1], Product3/1
  Dead Zone/1 -> Gain/1
  Fourier/2 -> Sum/1
  Fourier1/1 -> Saturation/1
  Sum1/1 -> Switch/1  "error"
  Constant2/1 -> Switch/3
  Trigonometric Function/1 -> Product2/2
  Gain/1 -> Discrete-Time Integrator/1
  Discrete-Time Integrator/1 -> Switch1/1
  Switch/1 -> Dead Zone/1
  Fourier1/2 -> Sum/2
  Constant3/1 -> Switch1/3
  deg-to-rad conversion/1 -> Trigonometric Function/1
  PV_Current/1 -> Mean/1, Fourier/1
  Product2/1 -> Sum1/1  "dI/dV (PV)"
  Saturation/1 -> Product/2
  Fourier/1 -> Product/1
  Switch1/1 -> delta D/1

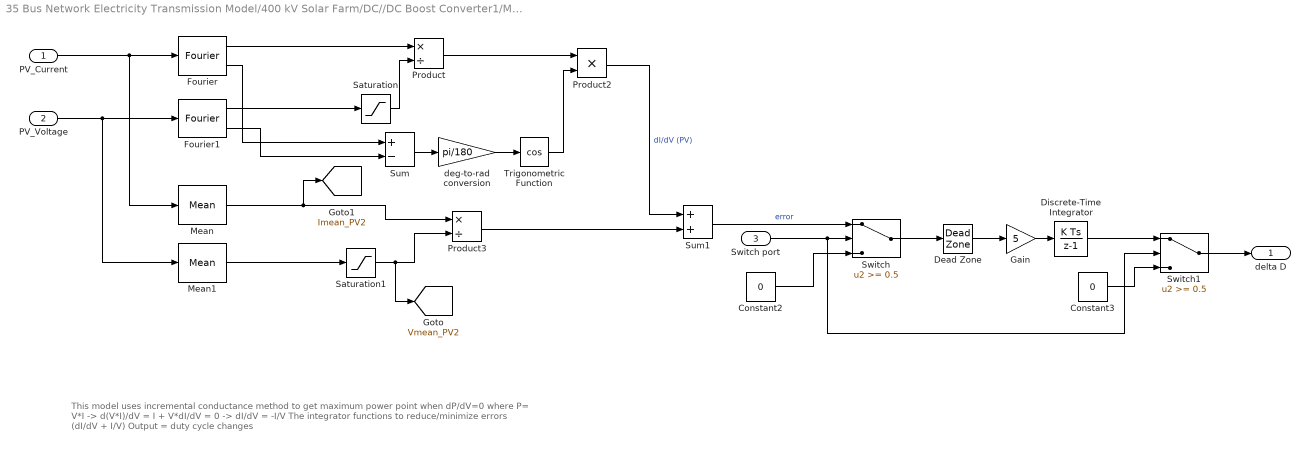
== system 35 Bus Network Electricity Transmission Model/400 kV Solar Farm/DC//DC Boost Converter1/MPPT/MPPT  ==
  note: This model uses incremental conductance method to get maximum power point
      |
      | when dP/dV=0  where P= V*I
      | -> d(V*I)/dV = I + V*dI/dV = 0
      | -> dI/dV = -I/V
      |
      | The integrator functions to reduce/minimize errors (dI/dV + I/V)
      | Output = duty cycle changes
  PV_Current : Inport
  PV_Voltage : Inport  Port=2
  Switch port : Inport  Port=3
  Constant2 : Constant  Value=0
  Constant3 : Constant  Value=0
  Dead Zone : DeadZone  LowerValue=-0.05  UpperValue=0.05
  Discrete-Time Integrator : DiscreteIntegrator  SampleTime=T_set  LimitOutput=on  UpperSaturationLimit=1  LowerSaturationLimit=-1  ICPrevOutput=DiscIntNeverNeededParam  ICPrevScaledInput=DiscIntNeverNeededParam
  Fourier : spsFourierLib/Fourier  Freq=1/(MPPT_time)  n=1  InInit=[0, 0]  Ts=T_set
  Fourier1 : spsFourierLib/Fourier  Freq=1/(MPPT_time)  n=1  InInit=[0, 0]  Ts=T_set
  Gain : Gain  Gain=5
  Mean : spsMeanLib/Mean  Freq=1/(MPPT_time)  Vinit=0  Ts=T_set
  Mean1 : spsMeanLib/Mean  Freq=1/(MPPT_time)  Vinit=0  Ts=T_set
  Product : Product  Inputs=*/
  Product2 : Product
  Product3 : Product  Inputs=*/
  Saturation : Saturate  UpperLimit=inf  LowerLimit=eps  ZeroCross=off
  Saturation1 : Saturate  UpperLimit=inf  LowerLimit=eps  ZeroCross=off
  Sum : Sum  Inputs=+-
  Sum1 : Sum
  Switch : Switch  Threshold=0.5  SaturateOnIntegerOverflow=off  InputSameDT=off
  Switch1 : Switch  Threshold=0.5  SaturateOnIntegerOverflow=off  InputSameDT=off
  Trigonometric Function : Trigonometry  Operator=cos
  deg-to-rad conversion : Gain  Gain=pi/180
  delta D : Outport
  tag scope: Imean_PV2=global, Vmean_PV2=global
  wires:
  Mean1/1 -> Saturation1/1
  PV_Voltage/1 -> Mean1/1, Fourier1/1
  Sum/1 -> deg-to-rad conversion/1
  Product/1 -> Product2/1
  Product3/1 -> Sum1/2
  Saturation1/1 -> [Vmean_PV2], Product3/2
  Switch port/1 -> Switch/2, Switch1/2
  Mean/1 -> [Imean_PV2], Product3/1
  Dead Zone/1 -> Gain/1
  Fourier/2 -> Sum/1
  Fourier1/1 -> Saturation/1
  Sum1/1 -> Switch/1  "error"
  Constant2/1 -> Switch/3
  Trigonometric Function/1 -> Product2/2
  Gain/1 -> Discrete-Time Integrator/1
  Discrete-Time Integrator/1 -> Switch1/1
  Switch/1 -> Dead Zone/1
  Fourier1/2 -> Sum/2
  Constant3/1 -> Switch1/3
  deg-to-rad conversion/1 -> Trigonometric Function/1
  PV_Current/1 -> Mean/1, Fourier/1
  Product2/1 -> Sum1/1  "dI/dV (PV)"
  Saturation/1 -> Product/2
  Fourier/1 -> Product/1
  Switch1/1 -> delta D/1

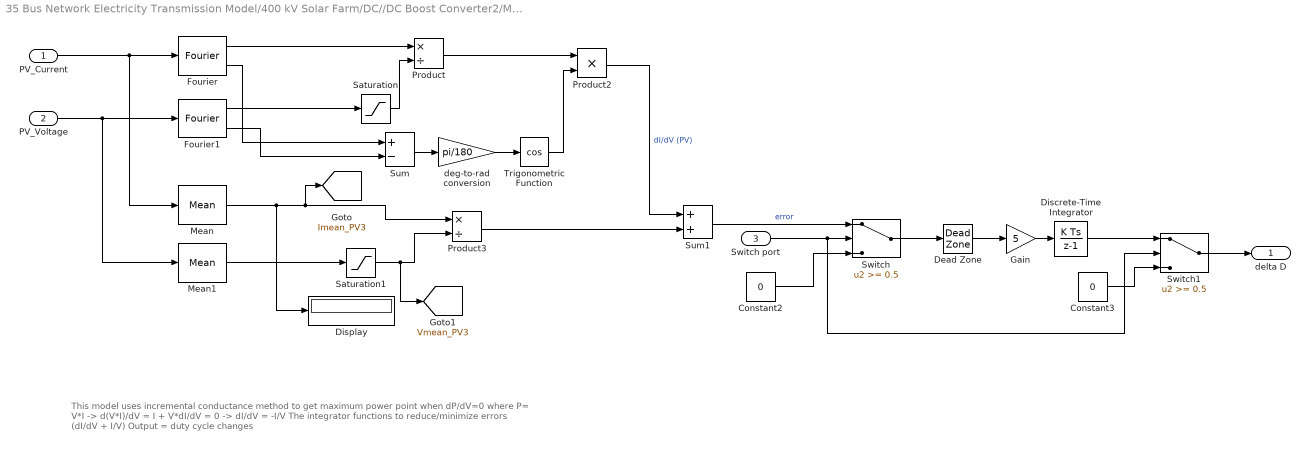
== system 35 Bus Network Electricity Transmission Model/400 kV Solar Farm/DC//DC Boost Converter2/MPPT/MPPT  ==
  note: This model uses incremental conductance method to get maximum power point
      |
      | when dP/dV=0  where P= V*I
      | -> d(V*I)/dV = I + V*dI/dV = 0
      | -> dI/dV = -I/V
      |
      | The integrator functions to reduce/minimize errors (dI/dV + I/V)
      | Output = duty cycle changes
  PV_Current : Inport
  PV_Voltage : Inport  Port=2
  Switch port : Inport  Port=3
  Constant2 : Constant  Value=0
  Constant3 : Constant  Value=0
  Dead Zone : DeadZone  LowerValue=-0.05  UpperValue=0.05
  Discrete-Time Integrator : DiscreteIntegrator  SampleTime=T_set  LimitOutput=on  UpperSaturationLimit=1  LowerSaturationLimit=-1  ICPrevOutput=DiscIntNeverNeededParam  ICPrevScaledInput=DiscIntNeverNeededParam
  Display : Display
  Fourier : spsFourierLib/Fourier  Freq=1/(MPPT_time)  n=1  InInit=[0, 0]  Ts=T_set
  Fourier1 : spsFourierLib/Fourier  Freq=1/(MPPT_time)  n=1  InInit=[0, 0]  Ts=T_set
  Gain : Gain  Gain=5
  Mean : spsMeanLib/Mean  Freq=1/(MPPT_time)  Vinit=0  Ts=T_set
  Mean1 : spsMeanLib/Mean  Freq=1/(MPPT_time)  Vinit=0  Ts=T_set
  Product : Product  Inputs=*/
  Product2 : Product
  Product3 : Product  Inputs=*/
  Saturation : Saturate  UpperLimit=inf  LowerLimit=eps  ZeroCross=off
  Saturation1 : Saturate  UpperLimit=inf  LowerLimit=eps  ZeroCross=off
  Sum : Sum  Inputs=+-
  Sum1 : Sum
  Switch : Switch  Threshold=0.5  SaturateOnIntegerOverflow=off  InputSameDT=off
  Switch1 : Switch  Threshold=0.5  SaturateOnIntegerOverflow=off  InputSameDT=off
  Trigonometric Function : Trigonometry  Operator=cos
  deg-to-rad conversion : Gain  Gain=pi/180
  delta D : Outport
  tag scope: Imean_PV3=global, Vmean_PV3=global
  wires:
  Mean1/1 -> Saturation1/1
  PV_Voltage/1 -> Mean1/1, Fourier1/1
  Sum/1 -> deg-to-rad conversion/1
  Product/1 -> Product2/1
  Product3/1 -> Sum1/2
  Saturation1/1 -> [Vmean_PV3], Product3/2
  Switch port/1 -> Switch/2, Switch1/2
  Dead Zone/1 -> Gain/1
  Fourier/2 -> Sum/1
  Fourier1/1 -> Saturation/1
  Sum1/1 -> Switch/1  "error"
  Constant2/1 -> Switch/3
  Trigonometric Function/1 -> Product2/2
  Gain/1 -> Discrete-Time Integrator/1
  Discrete-Time Integrator/1 -> Switch1/1
  Switch/1 -> Dead Zone/1
  Fourier1/2 -> Sum/2
  Constant3/1 -> Switch1/3
  deg-to-rad conversion/1 -> Trigonometric Function/1
  PV_Current/1 -> Mean/1, Fourier/1
  Product2/1 -> Sum1/1  "dI/dV (PV)"
  Saturation/1 -> Product/2
  Fourier/1 -> Product/1
  Switch1/1 -> delta D/1
  Mean/1 -> Display/1, [Imean_PV3], Product3/1

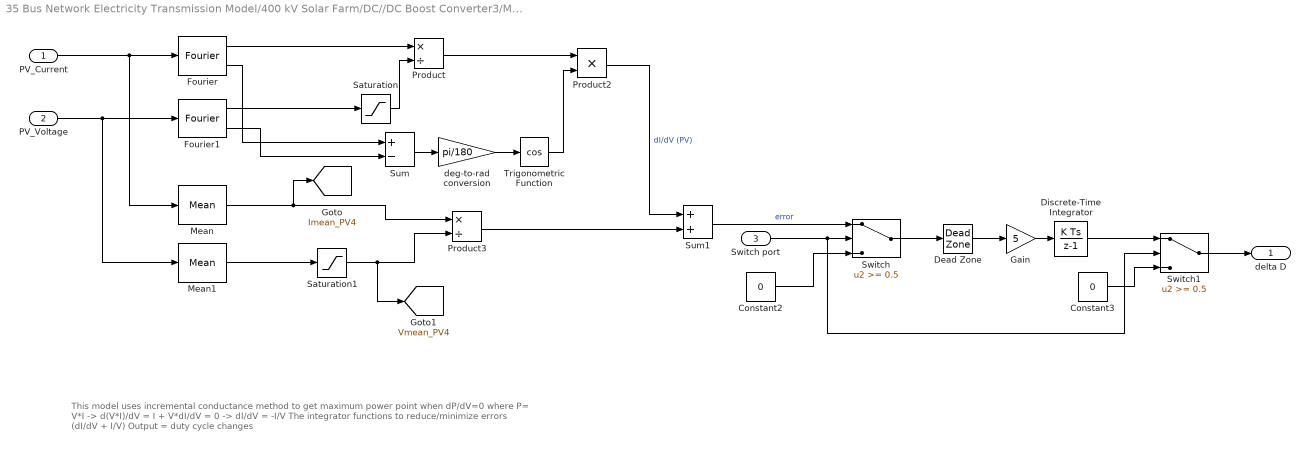
== system 35 Bus Network Electricity Transmission Model/400 kV Solar Farm/DC//DC Boost Converter3/MPPT/MPPT  ==
  note: This model uses incremental conductance method to get maximum power point
      |
      | when dP/dV=0  where P= V*I
      | -> d(V*I)/dV = I + V*dI/dV = 0
      | -> dI/dV = -I/V
      |
      | The integrator functions to reduce/minimize errors (dI/dV + I/V)
      | Output = duty cycle changes
  PV_Current : Inport
  PV_Voltage : Inport  Port=2
  Switch port : Inport  Port=3
  Constant2 : Constant  Value=0
  Constant3 : Constant  Value=0
  Dead Zone : DeadZone  LowerValue=-0.05  UpperValue=0.05
  Discrete-Time Integrator : DiscreteIntegrator  SampleTime=T_set  LimitOutput=on  UpperSaturationLimit=1  LowerSaturationLimit=-1  ICPrevOutput=DiscIntNeverNeededParam  ICPrevScaledInput=DiscIntNeverNeededParam
  Fourier : spsFourierLib/Fourier  Freq=1/(MPPT_time)  n=1  InInit=[0, 0]  Ts=T_set
  Fourier1 : spsFourierLib/Fourier  Freq=1/(MPPT_time)  n=1  InInit=[0, 0]  Ts=T_set
  Gain : Gain  Gain=5
  Mean : spsMeanLib/Mean  Freq=1/(MPPT_time)  Vinit=0  Ts=T_set
  Mean1 : spsMeanLib/Mean  Freq=1/(MPPT_time)  Vinit=0  Ts=T_set
  Product : Product  Inputs=*/
  Product2 : Product
  Product3 : Product  Inputs=*/
  Saturation : Saturate  UpperLimit=inf  LowerLimit=eps  ZeroCross=off
  Saturation1 : Saturate  UpperLimit=inf  LowerLimit=eps  ZeroCross=off
  Sum : Sum  Inputs=+-
  Sum1 : Sum
  Switch : Switch  Threshold=0.5  SaturateOnIntegerOverflow=off  InputSameDT=off
  Switch1 : Switch  Threshold=0.5  SaturateOnIntegerOverflow=off  InputSameDT=off
  Trigonometric Function : Trigonometry  Operator=cos
  deg-to-rad conversion : Gain  Gain=pi/180
  delta D : Outport
  tag scope: Imean_PV4=global, Vmean_PV4=global
  wires:
  Mean1/1 -> Saturation1/1
  PV_Voltage/1 -> Mean1/1, Fourier1/1
  Sum/1 -> deg-to-rad conversion/1
  Product/1 -> Product2/1
  Product3/1 -> Sum1/2
  Saturation1/1 -> [Vmean_PV4], Product3/2
  Switch port/1 -> Switch/2, Switch1/2
  Dead Zone/1 -> Gain/1
  Fourier/2 -> Sum/1
  Fourier1/1 -> Saturation/1
  Sum1/1 -> Switch/1  "error"
  Constant2/1 -> Switch/3
  Trigonometric Function/1 -> Product2/2
  Gain/1 -> Discrete-Time Integrator/1
  Discrete-Time Integrator/1 -> Switch1/1
  Switch/1 -> Dead Zone/1
  Fourier1/2 -> Sum/2
  Constant3/1 -> Switch1/3
  deg-to-rad conversion/1 -> Trigonometric Function/1
  PV_Current/1 -> Mean/1, Fourier/1
  Product2/1 -> Sum1/1  "dI/dV (PV)"
  Saturation/1 -> Product/2
  Fourier/1 -> Product/1
  Switch1/1 -> delta D/1
  Mean/1 -> [Imean_PV4], Product3/1

== system 35 Bus Network Electricity Transmission Model/North Network/Regulators 7/Turbine and Excitation Regulators/Stabilitator ==
  Pm : Inport
  Pe : Inport  Port=2
  dw : Inport  Port=3
  Add1 : Sum  Inputs=+-
  Generic Power System Stabilizer : spsGenericPowerSystemStabilizerLib/Generic Power System Stabilizer  Tsensor=30e-3  K=20  Twashout=2  Tleadlag1=[50e-3 20e-3]  Tleadlag2=[3 5.4]  VSlimits=[-0.15 0.15]  Vinit=0  Plot_On=off  MagdB_On=on  FreqRange=logspace(-2,2,500)
      settings: LibrarySourceBlock=|
      | sps_lib/Electrical Machines/Synchronous Machine Control/Generic
      | Power System Stabilizer
  Generic Power System Stabilizer1 : spsGenericPowerSystemStabilizerLib/Generic Power System Stabilizer  Tsensor=30e-3  K=20  Twashout=2  Tleadlag1=[50e-3 20e-3]  Tleadlag2=[3 5.4]  VSlimits=[-0.15 0.15]  Vinit=0  Plot_On=off  MagdB_On=on  FreqRange=logspace(-2,2,500)
      settings: LibrarySourceBlock=|
      | sps_lib/Electrical Machines/Synchronous Machine Control/Generic
      | Power System Stabilizer
  Ground : Ground
  Multiport Switch : MultiPortSwitch  DiagnosticForDefault=None  SaturateOnIntegerOverflow=off  InputSameDT=off
  Out1 : Outport
  wires:
  Pm/1 -> Add1/1
  Generic Power System Stabilizer1/1 -> Multiport Switch/4
  Pe/1 -> Add1/2
  Add1/1 -> Generic Power System Stabilizer/1
  Generic Power System Stabilizer/1 -> Multiport Switch/3
  dw/1 -> Generic Power System Stabilizer1/1
  Ground/1 -> Multiport Switch/2
  [PSS_modes] -> Multiport Switch/1
  Multiport Switch/1 -> Out1/1

== system 35 Bus Network Electricity Transmission Model/North Network/Regulators 8/Turbine and Excitation Regulators/Stabilitator ==
  Pm : Inport
  Pe : Inport  Port=2
  dw : Inport  Port=3
  Add1 : Sum  Inputs=+-
  Generic Power System Stabilizer : spsGenericPowerSystemStabilizerLib/Generic Power System Stabilizer  Tsensor=30e-3  K=20  Twashout=2  Tleadlag1=[50e-3 20e-3]  Tleadlag2=[3 5.4]  VSlimits=[-0.15 0.15]  Vinit=0  Plot_On=off  MagdB_On=on  FreqRange=logspace(-2,2,500)
      settings: LibrarySourceBlock=|
      | sps_lib/Electrical Machines/Synchronous Machine Control/Generic
      | Power System Stabilizer
  Generic Power System Stabilizer1 : spsGenericPowerSystemStabilizerLib/Generic Power System Stabilizer  Tsensor=30e-3  K=20  Twashout=2  Tleadlag1=[50e-3 20e-3]  Tleadlag2=[3 5.4]  VSlimits=[-0.15 0.15]  Vinit=0  Plot_On=off  MagdB_On=on  FreqRange=logspace(-2,2,500)
      settings: LibrarySourceBlock=|
      | sps_lib/Electrical Machines/Synchronous Machine Control/Generic
      | Power System Stabilizer
  Ground : Ground
  Multiport Switch : MultiPortSwitch  DiagnosticForDefault=None  SaturateOnIntegerOverflow=off  InputSameDT=off
  Out1 : Outport
  wires:
  Pm/1 -> Add1/1
  Generic Power System Stabilizer1/1 -> Multiport Switch/4
  Pe/1 -> Add1/2
  Add1/1 -> Generic Power System Stabilizer/1
  Generic Power System Stabilizer/1 -> Multiport Switch/3
  dw/1 -> Generic Power System Stabilizer1/1
  Ground/1 -> Multiport Switch/2
  [PSS_modes] -> Multiport Switch/1
  Multiport Switch/1 -> Out1/1

== system 35 Bus Network Electricity Transmission Model/North Network/Regulators 9/Turbine and Excitation Regulators/Stabilitator ==
  Pm : Inport
  Pe : Inport  Port=2
  dw : Inport  Port=3
  Add1 : Sum  Inputs=+-
  Generic Power System Stabilizer : spsGenericPowerSystemStabilizerLib/Generic Power System Stabilizer  Tsensor=30e-3  K=20  Twashout=2  Tleadlag1=[50e-3 20e-3]  Tleadlag2=[3 5.4]  VSlimits=[-0.15 0.15]  Vinit=0  Plot_On=off  MagdB_On=on  FreqRange=logspace(-2,2,500)
      settings: LibrarySourceBlock=|
      | sps_lib/Electrical Machines/Synchronous Machine Control/Generic
      | Power System Stabilizer
  Generic Power System Stabilizer1 : spsGenericPowerSystemStabilizerLib/Generic Power System Stabilizer  Tsensor=30e-3  K=20  Twashout=2  Tleadlag1=[50e-3 20e-3]  Tleadlag2=[3 5.4]  VSlimits=[-0.15 0.15]  Vinit=0  Plot_On=off  MagdB_On=on  FreqRange=logspace(-2,2,500)
      settings: LibrarySourceBlock=|
      | sps_lib/Electrical Machines/Synchronous Machine Control/Generic
      | Power System Stabilizer
  Ground : Ground
  Multiport Switch : MultiPortSwitch  DiagnosticForDefault=None  SaturateOnIntegerOverflow=off  InputSameDT=off
  Stab : Outport
  wires:
  Pm/1 -> Add1/1
  Generic Power System Stabilizer1/1 -> Multiport Switch/4
  Pe/1 -> Add1/2
  Add1/1 -> Generic Power System Stabilizer/1
  Generic Power System Stabilizer/1 -> Multiport Switch/3
  dw/1 -> Generic Power System Stabilizer1/1
  Ground/1 -> Multiport Switch/2
  [PSS_modes] -> Multiport Switch/1
  Multiport Switch/1 -> Stab/1

== system 35 Bus Network Electricity Transmission Model/South Network/Regulators 1/Turbine and Excitation Regulators/Stabilitator ==
  Pm : Inport
  Pe : Inport  Port=2
  dw : Inport  Port=3
  Add1 : Sum  Inputs=+-
  Generic Power System Stabilizer : spsGenericPowerSystemStabilizerLib/Generic Power System Stabilizer  Tsensor=30e-3  K=20  Twashout=2  Tleadlag1=[50e-3 20e-3]  Tleadlag2=[3 5.4]  VSlimits=[-0.15 0.15]  Vinit=0  Plot_On=off  MagdB_On=on  FreqRange=logspace(-2,2,500)
      settings: LibrarySourceBlock=|
      | sps_lib/Electrical Machines/Synchronous Machine Control/Generic
      | Power System Stabilizer
  Generic Power System Stabilizer1 : spsGenericPowerSystemStabilizerLib/Generic Power System Stabilizer  Tsensor=30e-3  K=20  Twashout=2  Tleadlag1=[50e-3 20e-3]  Tleadlag2=[3 5.4]  VSlimits=[-0.15 0.15]  Vinit=0  Plot_On=off  MagdB_On=on  FreqRange=logspace(-2,2,500)
      settings: LibrarySourceBlock=|
      | sps_lib/Electrical Machines/Synchronous Machine Control/Generic
      | Power System Stabilizer
  Ground : Ground
  Multiport Switch : MultiPortSwitch  DiagnosticForDefault=None  SaturateOnIntegerOverflow=off  InputSameDT=off
  Out1 : Outport
  wires:
  Pm/1 -> Add1/1
  Generic Power System Stabilizer1/1 -> Multiport Switch/4
  Pe/1 -> Add1/2
  Add1/1 -> Generic Power System Stabilizer/1
  Generic Power System Stabilizer/1 -> Multiport Switch/3
  dw/1 -> Generic Power System Stabilizer1/1
  Ground/1 -> Multiport Switch/2
  [PSS_modes] -> Multiport Switch/1
  Multiport Switch/1 -> Out1/1

== system 35 Bus Network Electricity Transmission Model/South Network/Regulators 2/Turbine and Excitation Regulators/Stabilitator ==
  Pm : Inport
  Pe : Inport  Port=2
  dw : Inport  Port=3
  Add1 : Sum  Inputs=+-
  Generic Power System Stabilizer : spsGenericPowerSystemStabilizerLib/Generic Power System Stabilizer  Tsensor=30e-3  K=20  Twashout=2  Tleadlag1=[50e-3 20e-3]  Tleadlag2=[3 5.4]  VSlimits=[-0.15 0.15]  Vinit=0  Plot_On=off  MagdB_On=on  FreqRange=logspace(-2,2,500)
      settings: LibrarySourceBlock=|
      | sps_lib/Electrical Machines/Synchronous Machine Control/Generic
      | Power System Stabilizer
  Generic Power System Stabilizer1 : spsGenericPowerSystemStabilizerLib/Generic Power System Stabilizer  Tsensor=30e-3  K=20  Twashout=2  Tleadlag1=[50e-3 20e-3]  Tleadlag2=[3 5.4]  VSlimits=[-0.15 0.15]  Vinit=0  Plot_On=off  MagdB_On=on  FreqRange=logspace(-2,2,500)
      settings: LibrarySourceBlock=|
      | sps_lib/Electrical Machines/Synchronous Machine Control/Generic
      | Power System Stabilizer
  Ground : Ground
  Multiport Switch : MultiPortSwitch  DiagnosticForDefault=None  SaturateOnIntegerOverflow=off  InputSameDT=off
  Out1 : Outport
  wires:
  Pm/1 -> Add1/1
  Generic Power System Stabilizer1/1 -> Multiport Switch/4
  Pe/1 -> Add1/2
  Add1/1 -> Generic Power System Stabilizer/1
  Generic Power System Stabilizer/1 -> Multiport Switch/3
  dw/1 -> Generic Power System Stabilizer1/1
  Ground/1 -> Multiport Switch/2
  [PSS_modes] -> Multiport Switch/1
  Multiport Switch/1 -> Out1/1

== system 35 Bus Network Electricity Transmission Model/South Network/Regulators 3/Turbine and Excitation Regulators/Stabilitator ==
  Pm : Inport
  Pe : Inport  Port=2
  dw : Inport  Port=3
  Add1 : Sum  Inputs=+-
  Generic Power System Stabilizer : spsGenericPowerSystemStabilizerLib/Generic Power System Stabilizer  Tsensor=30e-3  K=20  Twashout=2  Tleadlag1=[50e-3 20e-3]  Tleadlag2=[3 5.4]  VSlimits=[-0.15 0.15]  Vinit=0  Plot_On=off  MagdB_On=on  FreqRange=logspace(-2,2,500)
      settings: LibrarySourceBlock=|
      | sps_lib/Electrical Machines/Synchronous Machine Control/Generic
      | Power System Stabilizer
  Generic Power System Stabilizer1 : spsGenericPowerSystemStabilizerLib/Generic Power System Stabilizer  Tsensor=30e-3  K=20  Twashout=2  Tleadlag1=[50e-3 20e-3]  Tleadlag2=[3 5.4]  VSlimits=[-0.15 0.15]  Vinit=0  Plot_On=off  MagdB_On=on  FreqRange=logspace(-2,2,500)
      settings: LibrarySourceBlock=|
      | sps_lib/Electrical Machines/Synchronous Machine Control/Generic
      | Power System Stabilizer
  Ground : Ground
  Multiport Switch : MultiPortSwitch  DiagnosticForDefault=None  SaturateOnIntegerOverflow=off  InputSameDT=off
  Out1 : Outport
  wires:
  Pm/1 -> Add1/1
  Generic Power System Stabilizer1/1 -> Multiport Switch/4
  Pe/1 -> Add1/2
  Add1/1 -> Generic Power System Stabilizer/1
  Generic Power System Stabilizer/1 -> Multiport Switch/3
  dw/1 -> Generic Power System Stabilizer1/1
  Ground/1 -> Multiport Switch/2
  [PSS_modes] -> Multiport Switch/1
  Multiport Switch/1 -> Out1/1
